simulink model "Tutorial_8"  (R2022b)
settings: Solver=ode1  StartTime=0.0  StopTime=3  FixedStep=0.01  RelTol=1e-3
values from neighbouring files (symbols this model uses):
  b = 3750    [Tutorial8.m]
  F = 4500    [Tutorial8.m]
  Fg = F * g    (= 44145)    [Tutorial8.m]
  k = 220000    [Tutorial8.m]
  m = 450    [Tutorial8.m]
settings Model: Creator=manun  LastModifiedBy=manun

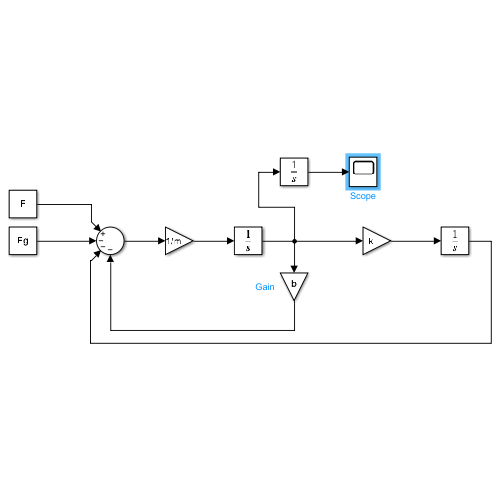
[thumbnail: Simulink's stored preview of the top-level diagram]
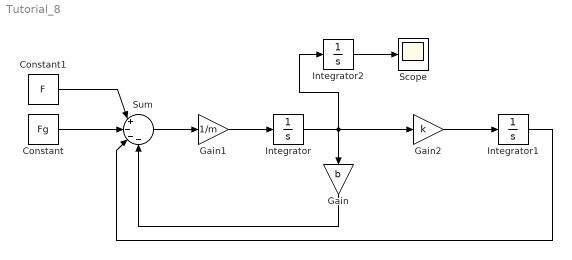
== system Tutorial_8 ==
  Constant : Constant  Value=Fg
  Constant1 : Constant  Value=F
  Gain : Gain  Gain=b
  Gain1 : Gain  Gain=1/m
  Gain2 : Gain  Gain=k
  Integrator : Integrator
  Integrator1 : Integrator
  Integrator2 : Integrator
  Scope : Scope
  Sum : Sum  Inputs=|+---
  wires:
  Sum/1 -> Gain1/1
  Integrator/1 -> Integrator2/1, Gain2/1, Gain/1
  Gain/1 -> Sum/4
  Integrator1/1 -> Sum/3
  Constant1/1 -> Sum/1
  Constant/1 -> Sum/2
  Gain1/1 -> Integrator/1
  Gain2/1 -> Integrator1/1
  Integrator2/1 -> Scope/1
